simulink model "rightcameraagent"  (Simulink 6.2)
settings: Solver=ode45  StartTime=0.0  StopTime=10.0  RelTol=1e-3
settings Model: LastModifiedBy=suarezjl
settings DataIOCC: SignalLoggingName=sigsOut
settings HardwareCC: TargetUnknown=on

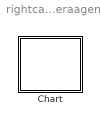
== system rightcameraagent ==
  Chart : Stateflow chart

== stateflow chart Chart ==
  state Initial
    \\Sally\LeftReachDemo\HeadModule\RightCameraAgent\FrameGrabber.Initialize()
    \\Sally\LeftReachDemo\HeadModule\RightCameraAgent\FrameGrabber.ObtainImage()
    \\Sally\LeftReachDemo\HeadModule\RightCameraAgent\FrameGrabber.ObtainImage()
    \\Sally\LeftReachDemo\HeadModule\RightCameraAgent\ColorSegmenter.Initial()
    \\Sally\LeftReachDemo\HeadModule\RightCameraAgent\ColorSegmenter.LoadColorModel()
  state Segmentation
    \\Sally\LeftReachDemo\HeadModule\RightCameraAgent\FrameGrabber.ObtainImage()
    \\Sally\LeftReachDemo\HeadModule\RightCameraAgent\ColorSegmenter.DoSegment()
  (default) -> Initial : Start
  Initial -> Segmentation : Always
  Segmentation -> Segmentation : Always
